simulink model "AdaptiveBackstepping"  (R2019b)
settings: Solver=ode23s  StartTime=0.0  StopTime=25  MaxStep=0.5  RelTol=1e-3  AbsTol=1e-6
undefined symbols (not defined in the file): a0, a1, a2, a3, dq0, Kd_endEff, lambda, parameter, Pi0, q0, R, x_endEff_D
libraries: simulink x1
settings Model: Creator=ariannagasparri  LastModifiedBy=ariannagasparri

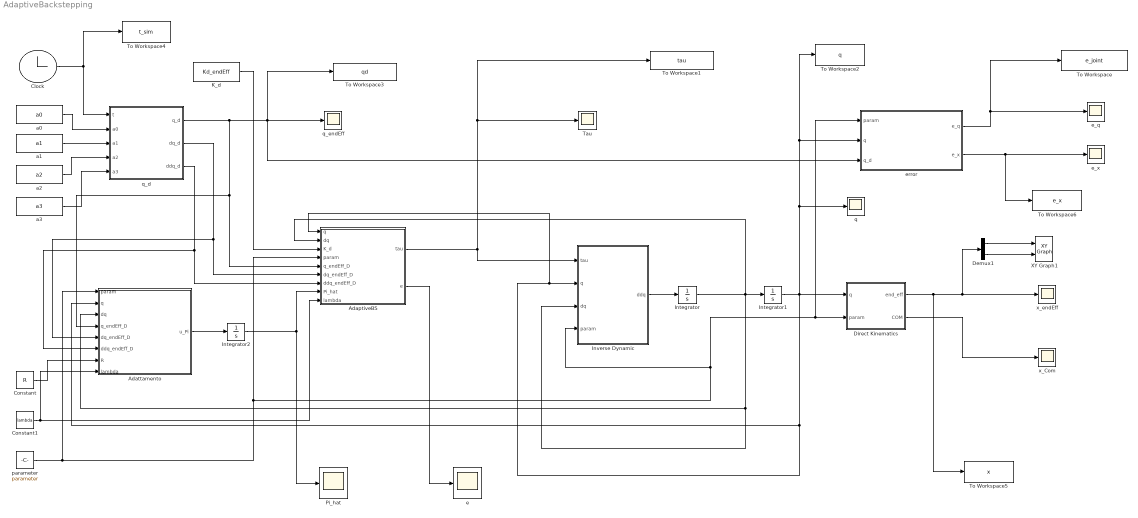
== system AdaptiveBackstepping ==
  AdaptiveBS : MATLAB Function  TreatAsAtomicUnit=on
  Adattamento : MATLAB Function  TreatAsAtomicUnit=on
  Clock : Clock
  Constant : Constant  Value=R
  Constant1 : Constant  Value=lambda
  Demux1 : Demux  Outputs=3
  "Direct Kinematics " : MATLAB Function  TreatAsAtomicUnit=on
  Integrator : Integrator  InitialCondition=q0
  Integrator1 : Integrator  InitialCondition=dq0
  Integrator2 : Integrator  InitialCondition=Pi0
  "Inverse Dynamic " : MATLAB Function  TreatAsAtomicUnit=on
  K_d : Constant  Value=Kd_endEff
  Pi_hat : Scope
  Tau : Scope
  To Workspace : ToWorkspace  VariableName=e_joint  SaveFormat=Structure With Time  SampleTime=-1
      settings: Save2DSignal=2-D array (concatenate along first dimension)
  To Workspace1 : ToWorkspace  VariableName=tau  SaveFormat=Structure With Time  SampleTime=-1
  To Workspace2 : ToWorkspace  VariableName=q  SaveFormat=Structure With Time  SampleTime=-1
  To Workspace3 : ToWorkspace  VariableName=qd  SaveFormat=Structure With Time  SampleTime=-1
  To Workspace4 : ToWorkspace  VariableName=t_sim  SaveFormat=Structure With Time  SampleTime=-1
  To Workspace5 : ToWorkspace  VariableName=x  SaveFormat=Structure With Time  SampleTime=-1
  To Workspace6 : ToWorkspace  VariableName=e_x  SaveFormat=Structure With Time  SampleTime=-1
  XY Graph1 : simulink/Sinks/XY Graph  xmin=x_endEff_D(1)-2  xmax=x_endEff_D(1)+2  ymin=x_endEff_D(3)-2  ymax=x_endEff_D(3)+2  st=-1
  a0 : Constant  Value=a0
  a1 : Constant  Value=a1
  a2 : Constant  Value=a2
  a3 : Constant  Value=a3
  e : Scope
  e_q : Scope
  e_x : Scope
  error : MATLAB Function  TreatAsAtomicUnit=on
  "parameter " : Constant  Value=parameter
  q : Scope
  q_d : MATLAB Function  TreatAsAtomicUnit=on
  q_endEff : Scope
  x_Com : Scope
  x_endEff : Scope
  wires:
  "Direct Kinematics "/1(end_eff) -> To Workspace5/1, Demux1/1, x_endEff/1
  error/1(e_q) -> To Workspace/1, e_q/1
  "Direct Kinematics "/2(COM) -> x_Com/1
  Demux1/3 -> XY Graph1/2
  a2/1 -> q_d/4(a2)
  Integrator1/1 -> "Direct Kinematics "/1(q), To Workspace2/1, error/2(q), q/1, Adattamento/2(q), AdaptiveBS/1(q), "Inverse Dynamic "/2(q)
  a3/1 -> q_d/5(a3)
  error/2(e_x) -> To Workspace6/1, e_x/1
  "parameter "/1 -> Adattamento/1(param), AdaptiveBS/4(param), "Inverse Dynamic "/4(param), error/1(param), "Direct Kinematics "/2(param)
  a1/1 -> q_d/3(a1)
  Integrator/1 -> AdaptiveBS/2(dq), Adattamento/3(dq), "Inverse Dynamic "/3(dq), Integrator1/1
  q_d/1(q_d) -> Adattamento/4(q_endEff_D), AdaptiveBS/5(q_endEff_D), error/3(q_d), To Workspace3/1, q_endEff/1
  "Inverse Dynamic "/1(ddq) -> Integrator/1
  AdaptiveBS/2(e) -> e/1
  a0/1 -> q_d/2(a0)
  Clock/1 -> q_d/1(t), To Workspace4/1
  Demux1/1 -> XY Graph1/1
  K_d/1 -> AdaptiveBS/3(K_d)
  Adattamento/1(u_Pi) -> Integrator2/1
  q_d/2(dq_d) -> Adattamento/5(dq_endEff_D), AdaptiveBS/6(dq_endEff_D)
  q_d/3(ddq_d) -> Adattamento/6(ddq_endEff_D), AdaptiveBS/7(ddq_endEff_D)
  Integrator2/1 -> Pi_hat/1, AdaptiveBS/8(Pi_hat)
  Constant/1 -> Adattamento/7(R)
  Constant1/1 -> AdaptiveBS/9(lambda), Adattamento/8(lambda)
  AdaptiveBS/1(tau) -> To Workspace1/1, Tau/1, "Inverse Dynamic "/1(tau)

== matlab function AdaptiveBackstepping/Direct Kinematics  ==
  data: q input; end_eff output; param input; COM output
function [end_eff, COM] = DirectK(q,param)

    [Pcom, Etip, ~, ~, ~, ~, ~, ~, ~] =  forwardKinematics(param, q);
    
    end_eff = Etip(1:3, 4);
    COM = Pcom;
    
end

== matlab function AdaptiveBackstepping/Inverse Dynamic  ==
  data: tau input; q input; dq input; ddq output; param input
function ddq = inverseDynamic(tau, q, dq, param)

    B = B_fun(param, q);
    C = C_fun(param, q, dq);
    G = G_fun(param, q);
    
    ddq = pinv(B)*(tau - G - C*dq);

end

== matlab function AdaptiveBackstepping/AdaptiveBS ==
  data: q input; tau output; dq input; K_d input; param input; q_endEff_D input; dq_endEff_D input; e output; ddq_endEff_D input; Pi_hat input; lambda input
function [tau, e]  = x_now(q, dq, K_d, param, q_endEff_D, dq_endEff_D, ddq_endEff_D, Pi_hat, lambda)

    Y = Y_fun(param, q, dq, ddq_endEff_D);
    
    [Pcom, Etip] = forwardKinematics(param, q_endEff_D);
    x_endEff_D = Etip(1:3, 4);
    [Pcom, Etip] = forwardKinematics(param, q);
    x = Etip(1:3, 4);
    J = JacobianEndEff(param, q);
    dx_endEff_D = J * dq_endEff_D;
    dx = J * dq;

    e = x_endEff_D - x;
    de = dx_endEff_D - dx;
    
    s = pinv(J) * (de + lambda * e);
    
    tau = Y * Pi_hat + K_d * s + J' * e;

end

== matlab function AdaptiveBackstepping/error ==
  data: param input; q input; e_q output; q_d input; e_x output
function [e_q, e_x]  = error(param, q, q_d)
    

    [~, Etip, ~, ~, ~, ~, ~, ~, ~] =  forwardKinematics(param, q);
    [~, Etip_d, ~, ~, ~, ~, ~, ~, ~] =  forwardKinematics(param, q_d);  

    e_x = Etip_d(1:3,4) - Etip(1:3,4);

    e_q = q_d - q;
    
end

== matlab function AdaptiveBackstepping/q_d ==
  data: t input; q_d output; dq_d output; ddq_d output; a0 input; a1 input; a2 input; a3 input
function [q_d, dq_d, ddq_d] = desiderable_q(t, a0, a1, a2, a3)

    [q_d, dq_d, ddq_d] = vettoreq(a0, a1, a2, a3, t);
    
end

== matlab function AdaptiveBackstepping/Adattamento ==
  data: param input; q input; dq input; q_endEff_D input; dq_endEff_D input; ddq_endEff_D input; u_Pi output; R input; lambda input
function u_Pi = adattamento(param, q, dq, q_endEff_D, dq_endEff_D, ddq_endEff_D, R, lambda)

    Y = Y_fun(param, q, dq, ddq_endEff_D);

    [Pcom, Etip] = forwardKinematics(param, q_endEff_D);
    x_endEff_D = Etip(1:3,4);
    [Pcom, Etip] = forwardKinematics(param, q);
    x = Etip(1:3,4);
    J = JacobianEndEff(param, q);
    dx_endEff_D = J * dq_endEff_D;
    dx = J * dq;

    e = x_endEff_D - x;
    de = dx_endEff_D - dx;

    s = pinv(J) * (de + lambda * e);

    u_Pi = pinv(R) * Y' * s;

end
